simulink model "diobs_R23"  (R2023a)
settings: Solver=VariableStepAuto  StartTime=0.0  StopTime=0.2  RelTol=1e-3
values from neighbouring files (symbols this model uses):
  Adso = eye(2) + Aso * ts    [init_diobs.m]
  Cso = [1 0]    [init_diobs.m]
  komega = Ldso(2) / ts    [init_diobs.m]
  komega2 = Ldso2(2) / ts    [init_diobs.m]
  ktheta = Ldso(1) / ts    [init_diobs.m]
  ktheta2 = Ldso2(1) / ts    [init_diobs.m]
  Ldso = (acker(Adso',Cso',p2placed))'    [init_diobs.m]
  Ldso2 = (acker(Adso',Cso',p2placed))'    [init_diobs.m]
  omega_nom = 2*pi*50    (= 314.159265359)    [init_diobs.m]
  ts = 1e-4    (= 0.0001)    [init_diobs.m]
settings Model: Creator=dbagn  LastModifiedBy=ltnbda
settings RTWCC: GPUComputeCapability=5.0
settings ConfigComp: CovBoundaryAbsTol=1.0e-5

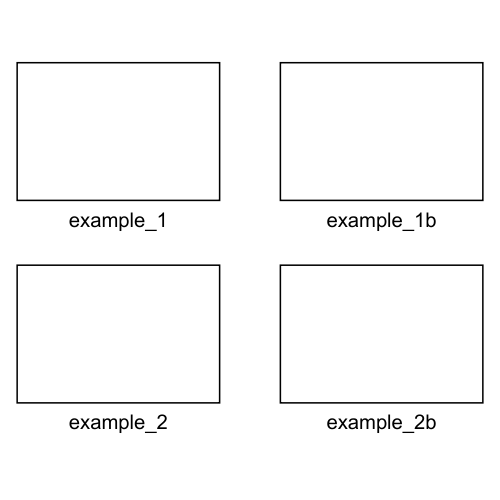
[thumbnail: Simulink's stored preview of the top-level diagram]
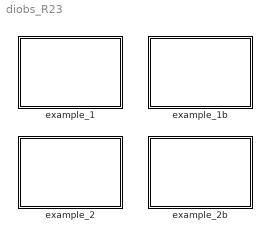
== system diobs_R23 ==
  example_1 : Subsystem
  example_1b : Subsystem
  example_2 : Subsystem
  example_2b : Subsystem

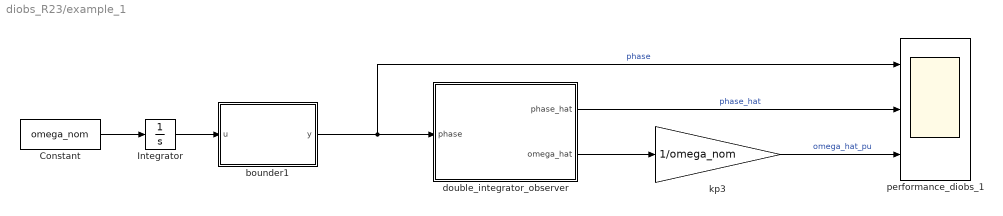
== system diobs_R23/example_1 ==
  Constant : Constant  Value=omega_nom
  Integrator : Integrator
  bounder1 : MATLAB Function  TreatAsAtomicUnit=on
  double_integrator_observer : Subsystem
  kp3 : Gain  Gain=1/omega_nom  SaturateOnIntegerOverflow=on  OutDataTypeStr=Inherit: Same as input  ParamDataTypeStr=Inherit: Same as input
  performance_diobs_1 : Scope  NumInputPorts=3
  wires:
  double_integrator_observer/1(phase_hat) -> performance_diobs_1/2  "phase_hat"
  kp3/1 -> performance_diobs_1/3  "omega_hat_pu"
  bounder1/1(y) -> double_integrator_observer/1(phase), performance_diobs_1/1  "phase"
  Constant/1 -> Integrator/1
  Integrator/1 -> bounder1/1(u)
  double_integrator_observer/2(omega_hat) -> kp3/1

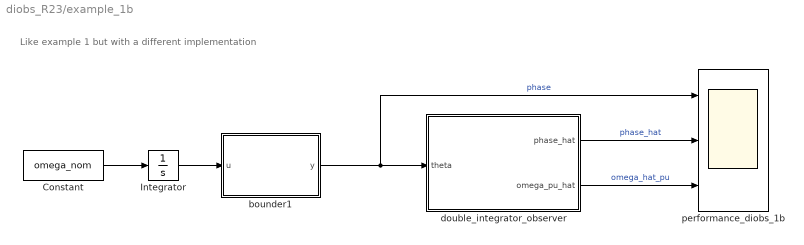
== system diobs_R23/example_1b ==
  note: Like example 1 but with a different implementation
  Constant : Constant  Value=omega_nom
  Integrator : Integrator
  bounder1 : MATLAB Function  TreatAsAtomicUnit=on
  double_integrator_observer : Subsystem
  performance_diobs_1b : Scope  NumInputPorts=3
  wires:
  Integrator/1 -> bounder1/1(u)
  Constant/1 -> Integrator/1
  bounder1/1(y) -> performance_diobs_1b/1, double_integrator_observer/1(theta)  "phase"
  double_integrator_observer/2(omega_pu_hat) -> performance_diobs_1b/3  "omega_hat_pu"
  double_integrator_observer/1(phase_hat) -> performance_diobs_1b/2  "phase_hat"

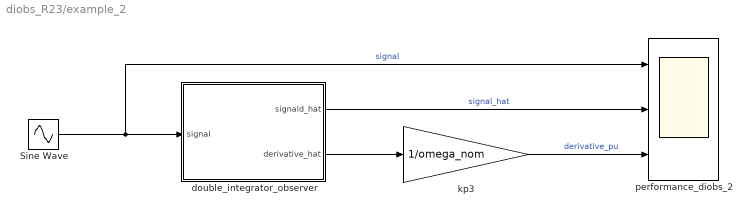
== system diobs_R23/example_2 ==
  Sine Wave : Sin  Frequency=omega_nom  SampleTime=0
  double_integrator_observer : Subsystem
  kp3 : Gain  Gain=1/omega_nom  SaturateOnIntegerOverflow=on  OutDataTypeStr=Inherit: Same as input  ParamDataTypeStr=Inherit: Same as input
  performance_diobs_2 : Scope  NumInputPorts=3
  wires:
  double_integrator_observer/2(derivative_hat) -> kp3/1
  Sine Wave/1 -> performance_diobs_2/1, double_integrator_observer/1(signal)  "signal"
  kp3/1 -> performance_diobs_2/3  "derivative_pu"
  double_integrator_observer/1(signald_hat) -> performance_diobs_2/2  "signal_hat"

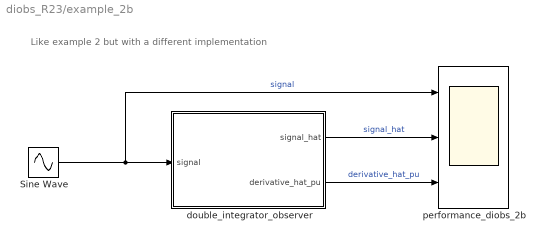
== system diobs_R23/example_2b ==
  note: Like example 2 but with a different implementation
  Sine Wave : Sin  Frequency=omega_nom  SampleTime=0
  double_integrator_observer : Subsystem
  performance_diobs_2b : Scope  NumInputPorts=3
  wires:
  double_integrator_observer/1(signal_hat) -> performance_diobs_2b/2  "signal_hat"
  double_integrator_observer/2(derivative_hat_pu) -> performance_diobs_2b/3  "derivative_hat_pu"
  Sine Wave/1 -> double_integrator_observer/1(signal), performance_diobs_2b/1  "signal"

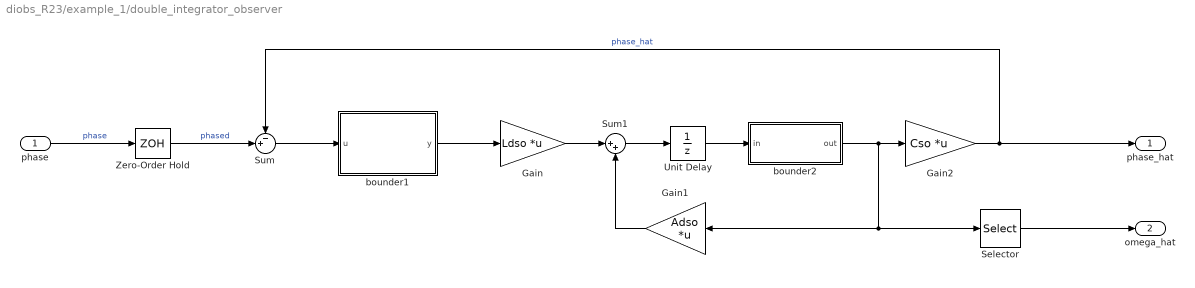
== system diobs_R23/example_1/double_integrator_observer ==
  phase : Inport
  Gain : Gain  Gain=Ldso  Multiplication=Matrix(K*u)
  Gain1 : Gain  Gain=Adso  Multiplication=Matrix(K*u)
  Gain2 : Gain  Gain=Cso  Multiplication=Matrix(K*u)
  Selector : Selector  InputPortWidth=2  IndexOptions=Index vector (dialog)  Indices=2  OutputSizes=1
  Sum : Sum  Inputs=-+|
  Sum1 : Sum  Inputs=|++
  Unit Delay : UnitDelay  SampleTime=-1  HasFrameUpgradeWarning=on
  Zero-Order Hold : ZeroOrderHold  SampleTime=ts
  bounder1 : MATLAB Function  TreatAsAtomicUnit=on
  bounder2 : Subsystem
  phase_hat : Outport
  omega_hat : Outport  Port=2
  wires:
  Gain/1 -> Sum1/1
  Selector/1 -> omega_hat/1
  Gain1/1 -> Sum1/2
  Sum1/1 -> Unit Delay/1
  Sum/1 -> bounder1/1(u)
  phase/1 -> Zero-Order Hold/1  "phase"
  bounder1/1(y) -> Gain/1
  Gain2/1 -> phase_hat/1, Sum/1  "phase_hat"
  Zero-Order Hold/1 -> Sum/2  "phased"
  Unit Delay/1 -> bounder2/1(in)
  bounder2/1(out) -> Selector/1, Gain1/1, Gain2/1

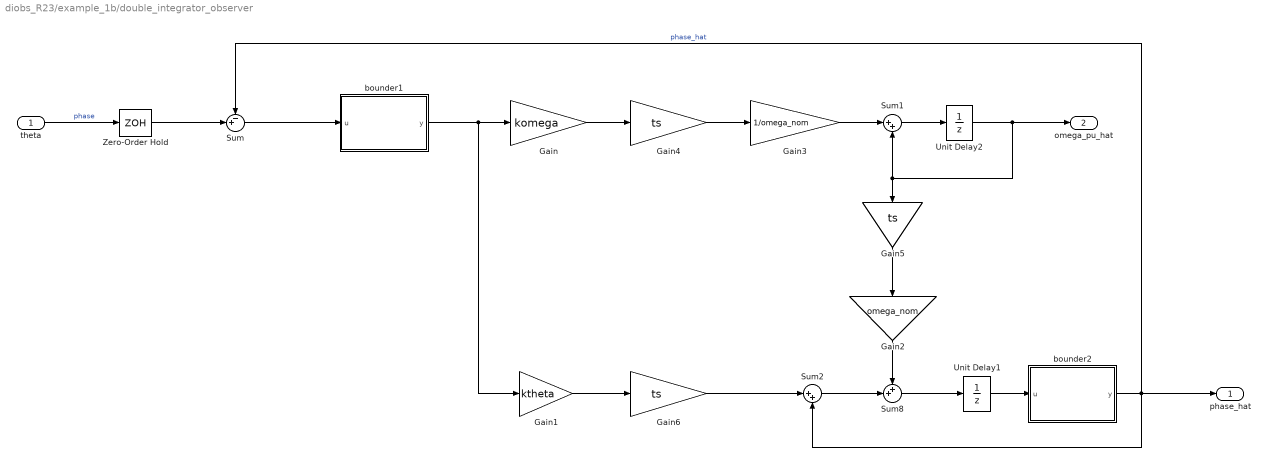
== system diobs_R23/example_1b/double_integrator_observer ==
  theta : Inport
  Gain : Gain  Gain=komega
  Gain1 : Gain  Gain=ktheta
  Gain2 : Gain  Gain=omega_nom
  Gain3 : Gain  Gain=1/omega_nom
  Gain4 : Gain  Gain=ts
  Gain5 : Gain  Gain=ts
  Gain6 : Gain  Gain=ts
  Sum : Sum  Inputs=-+|
  Sum1 : Sum  Inputs=|++
  Sum2 : Sum  Inputs=|++
  Sum8 : Sum  Inputs=++|
  Unit Delay1 : UnitDelay  SampleTime=-1  HasFrameUpgradeWarning=on
  Unit Delay2 : UnitDelay  SampleTime=-1  HasFrameUpgradeWarning=on
  Zero-Order Hold : ZeroOrderHold  SampleTime=ts
  bounder1 : MATLAB Function  TreatAsAtomicUnit=on
  bounder2 : MATLAB Function  TreatAsAtomicUnit=on
  phase_hat : Outport  VectorParamsAs1DForOutWhenUnconnected=off
  omega_pu_hat : Outport  Port=2  VectorParamsAs1DForOutWhenUnconnected=off
  wires:
  Gain1/1 -> Gain6/1
  theta/1 -> Zero-Order Hold/1  "phase"
  Sum8/1 -> Unit Delay1/1
  Unit Delay1/1 -> bounder2/1(u)
  Sum1/1 -> Unit Delay2/1
  Gain/1 -> Gain4/1
  Unit Delay2/1 -> omega_pu_hat/1, Sum1/2, Gain5/1
  Sum2/1 -> Sum8/2
  bounder2/1(y) -> Sum2/2, phase_hat/1, Sum/1  "phase_hat"
  bounder1/1(y) -> Gain1/1, Gain/1
  Gain2/1 -> Sum8/1
  Gain3/1 -> Sum1/1
  Gain5/1 -> Gain2/1
  Sum/1 -> bounder1/1(u)
  Gain4/1 -> Gain3/1
  Gain6/1 -> Sum2/1
  Zero-Order Hold/1 -> Sum/2

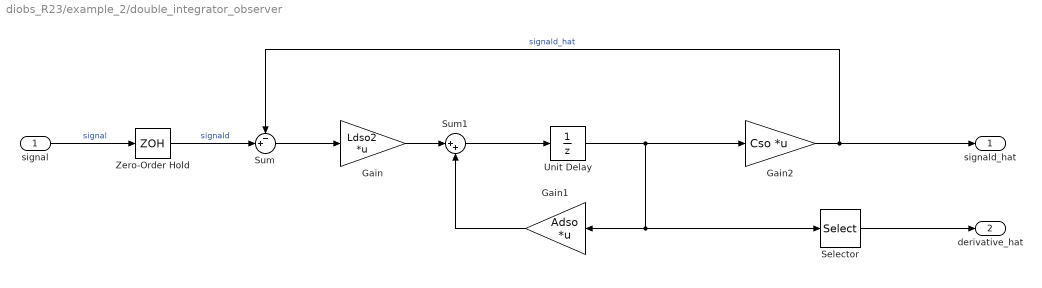
== system diobs_R23/example_2/double_integrator_observer ==
  signal : Inport
  Gain : Gain  Gain=Ldso2  Multiplication=Matrix(K*u)
  Gain1 : Gain  Gain=Adso  Multiplication=Matrix(K*u)
  Gain2 : Gain  Gain=Cso  Multiplication=Matrix(K*u)
  Selector : Selector  InputPortWidth=2  IndexOptions=Index vector (dialog)  Indices=2  OutputSizes=1
  Sum : Sum  Inputs=-+|
  Sum1 : Sum  Inputs=|++
  Unit Delay : UnitDelay  SampleTime=-1  HasFrameUpgradeWarning=on
  Zero-Order Hold : ZeroOrderHold  SampleTime=ts
  signald_hat : Outport
  derivative_hat : Outport  Port=2
  wires:
  Unit Delay/1 -> Gain2/1, Selector/1, Gain1/1
  Zero-Order Hold/1 -> Sum/2  "signald"
  Gain2/1 -> Sum/1, signald_hat/1  "signald_hat"
  Sum/1 -> Gain/1
  signal/1 -> Zero-Order Hold/1  "signal"
  Sum1/1 -> Unit Delay/1
  Gain1/1 -> Sum1/2
  Selector/1 -> derivative_hat/1
  Gain/1 -> Sum1/1

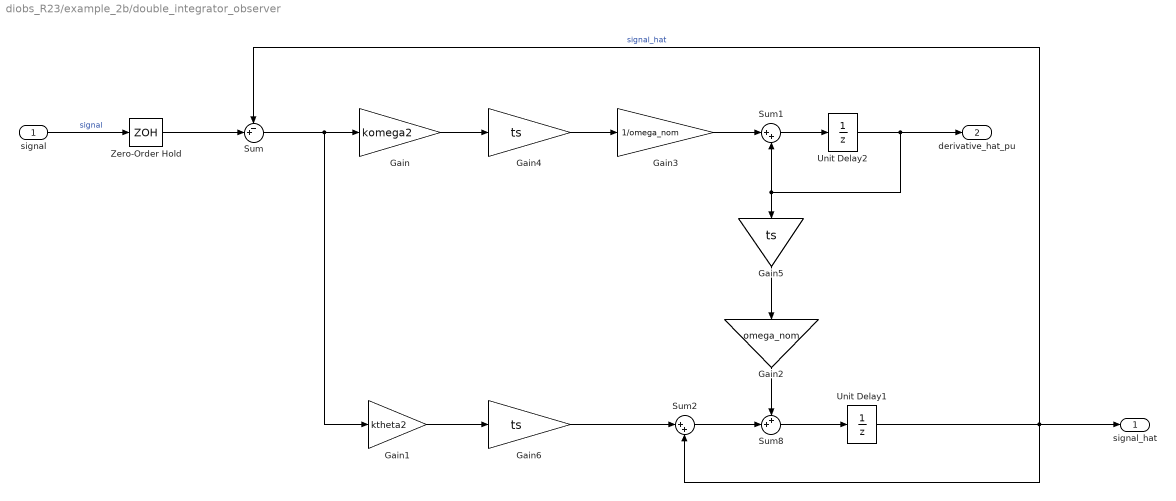
== system diobs_R23/example_2b/double_integrator_observer ==
  signal : Inport
  Gain : Gain  Gain=komega2
  Gain1 : Gain  Gain=ktheta2
  Gain2 : Gain  Gain=omega_nom
  Gain3 : Gain  Gain=1/omega_nom
  Gain4 : Gain  Gain=ts
  Gain5 : Gain  Gain=ts
  Gain6 : Gain  Gain=ts
  Sum : Sum  Inputs=-+|
  Sum1 : Sum  Inputs=|++
  Sum2 : Sum  Inputs=|++
  Sum8 : Sum  Inputs=++|
  Unit Delay1 : UnitDelay  SampleTime=-1  HasFrameUpgradeWarning=on
  Unit Delay2 : UnitDelay  SampleTime=-1  HasFrameUpgradeWarning=on
  Zero-Order Hold : ZeroOrderHold  SampleTime=ts
  signal_hat : Outport  VectorParamsAs1DForOutWhenUnconnected=off
  derivative_hat_pu : Outport  Port=2  VectorParamsAs1DForOutWhenUnconnected=off
  wires:
  Zero-Order Hold/1 -> Sum/2
  Gain6/1 -> Sum2/1
  Gain4/1 -> Gain3/1
  Gain5/1 -> Gain2/1
  Gain3/1 -> Sum1/1
  Gain2/1 -> Sum8/1
  Sum/1 -> Gain/1, Gain1/1
  Unit Delay1/1 -> Sum/1, signal_hat/1, Sum2/2  "signal_hat"
  Sum2/1 -> Sum8/2
  Unit Delay2/1 -> Gain5/1, Sum1/2, derivative_hat_pu/1
  Gain/1 -> Gain4/1
  Sum1/1 -> Unit Delay2/1
  Sum8/1 -> Unit Delay1/1
  signal/1 -> Zero-Order Hold/1  "signal"
  Gain1/1 -> Gain6/1

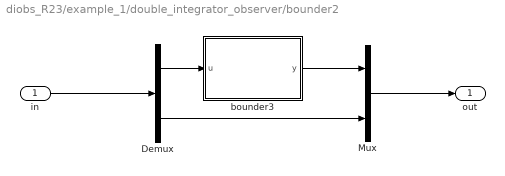
== system diobs_R23/example_1/double_integrator_observer/bounder2 ==
  in : Inport
  Demux : Demux  Outputs=2
  Mux : Mux  Inputs=2
  bounder3 : MATLAB Function  TreatAsAtomicUnit=on
  out : Outport
  wires:
  in/1 -> Demux/1
  Demux/1 -> bounder3/1(u)
  bounder3/1(y) -> Mux/1
  Demux/2 -> Mux/2
  Mux/1 -> out/1

== matlab function diobs_R23/example_1/bounder1 ==
  data: u input; y output
function y = bounder(u)
    
    y = -pi + mod(u+3*pi,2*pi);
    
end

== matlab function diobs_R23/example_1/double_integrator_observer/bounder2/bounder3 ==
  data: u input; y output
function y = bounder(u)
    
    y = -pi + mod(u+3*pi,2*pi);
    
end

== matlab function diobs_R23/example_1b/bounder1 ==
  data: u input; y output
function y = bounder(u)
    
    y = -pi + mod(u+3*pi,2*pi);
    
end

== matlab function diobs_R23/example_1/double_integrator_observer/bounder1 ==
  data: u input; y output
function y = bounder(u)
    
    y = -pi + mod(u+3*pi,2*pi);
    
end

== matlab function diobs_R23/example_1b/double_integrator_observer/bounder1 ==
  data: u input; y output
function y = bounder(u)
    
    y = -pi + mod(u+3*pi,2*pi);
end

== matlab function diobs_R23/example_1b/double_integrator_observer/bounder2 ==
  data: u input; y output
function y = bounder(u)
    
    u = -pi + mod(u+3*pi,2*pi);
    
    y = u;
end
